simulink model "acc_num6"  (R2020a)
settings: Solver=ode4  StartTime=0.0  StopTime=endt  FixedStep=0.002  RelTol=1e-3  EnableMultiTasking=on
values from neighbouring files (symbols this model uses):
  Dy = 0.0085    [acc_parameter_num6.m]
  Jy = J_body + 2*J_prop + J_yoke    (= 0.0219920648283)    [acc_parameter_num6.m]
  K_A = 30    [acc_parameter_num6.m]
  K_B = 300    [acc_parameter_num6.m]
  Kd = 10    [acc_parameter_num6.m]
  lead_id = [1,2]    [acc_parameter_num6.m]
  pos_base = [x0;y0]    [acc_parameter_num6.m]
  psi_initial = [pi*3/4,pi/4,pi/4,pi/4,pi*5/6,pi*4/5]    [acc_parameter_num6.m]
  target = [10;33]    [acc_parameter_num6.m]
libraries: simulink_extras x6, aerolibanimutils x1, dspnetwork x1
settings Model: ExtModeTrigDuration=10000  Creator=Aline  LastModifiedBy=Aline
settings SolverCC: PositivePriorityOrder=on
settings DataIOCC: ReturnWorkspaceOutputs=off
settings OptimizationCC: LifeSpan=inf
settings DebuggingCC: ArithmeticOperatorsInVariantConditions=warning
settings SFSimCC: SimUseLocalCustomCode=off  CustomCodeUndefinedFunction=UseInterfaceOnly
settings RTWCC: Description=QUARC Win64 Target  SystemTargetFile=quarc_win64.tlc  TemplateMakefile=quarc_default_tmf  RTWUseLocalCustomCode=off
settings CodeAppCC: StateflowObjectComments=on
settings STFCustomTargetCC: TargetPreCompLibLocation=C:\PROGRA~3\QUARC\lib\2020a\win64\release  TargetLangStandard=C99 (ISO)  ConcurrentExecutionCompliant=on  GRTInterface=on  SystemTargetFile=quarc_win64.tlc
settings GRTTargetCC: TargetPreCompLibLocation=C:\PROGRA~3\QUARC\lib\2020a\win64\release  ParMdlRefBuildCompliant=off  CompOptLevelCompliant=off  CombineOutputUpdateFcns=off  MatFileLogging=off  CPPClassGenCompliant=off  GRTInterface=on  UseToolchainInfoCompliant=off  ExtMode=on  ExtModeMexFile=quarc_comm
settings ConfigComp: CovMetricSettings=dswe

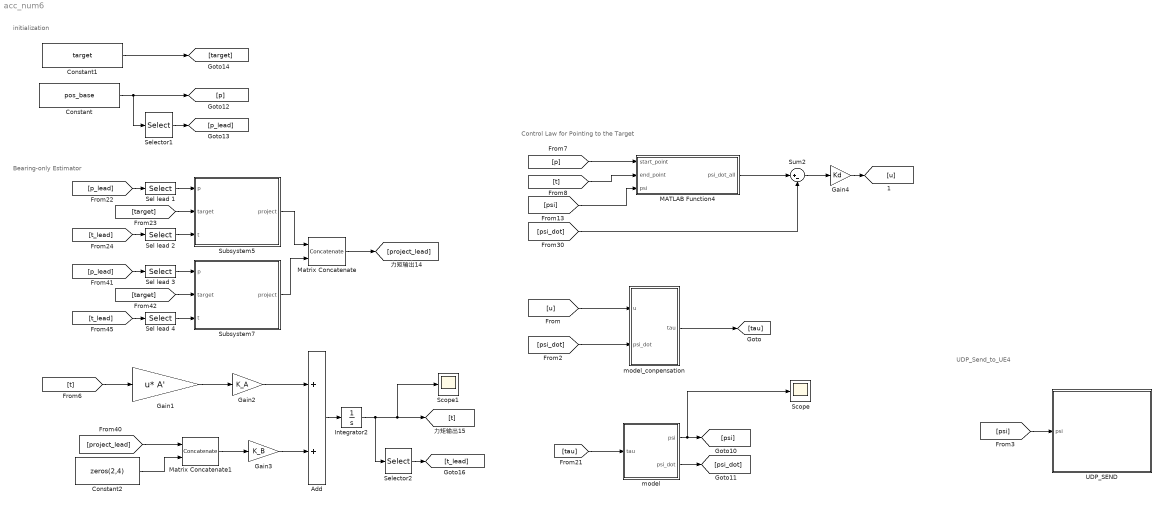
== system acc_num6 ==
  note: initialization
  note: Control Law for Pointing to the Target
  note: Bearing-only Estimator
  note: UDP_Send_to_UE4
  Add : Sum
  Constant : Constant  Value=pos_base
  Constant1 : Constant  Value=target  VectorParams1D=off
  Constant2 : Constant  Value=zeros(2,4)
  Gain1 : Gain  Gain=A'  Multiplication=Matrix(u*K)
  Gain2 : Gain  Gain=K_A
  Gain3 : Gain  Gain=K_B
  Gain4 : Gain  Gain=Kd
  Integrator2 : Integrator  InitialCondition=pos_base+ones(2,6)
  MATLAB Function4 : MATLAB Function  TreatAsAtomicUnit=on
  Matrix Concatenate : Concatenate  Mode=Multidimensional array  ConcatenateDimension=2
  Matrix Concatenate1 : Concatenate  Mode=Multidimensional array  ConcatenateDimension=2
  Scope : Scope
  Scope1 : Scope
  Sel lead 1 : Selector  NumberOfDimensions=2  InputPortWidth=3  IndexOptions=Index vector (dialog),Index vector (dialog)  Indices=[1 2],1  OutputSizes=1,1
  Sel lead 2 : Selector  NumberOfDimensions=2  InputPortWidth=3  IndexOptions=Index vector (dialog),Index vector (dialog)  Indices=[1 2],1  OutputSizes=1,1
  Sel lead 3 : Selector  NumberOfDimensions=2  InputPortWidth=3  IndexOptions=Index vector (dialog),Index vector (dialog)  Indices=[1 2],2  OutputSizes=1,1
  Sel lead 4 : Selector  NumberOfDimensions=2  InputPortWidth=3  IndexOptions=Index vector (dialog),Index vector (dialog)  Indices=[1 2],2  OutputSizes=1,1
  Selector1 : Selector  NumberOfDimensions=2  InputPortWidth=3  IndexOptions=Index vector (dialog),Index vector (dialog)  Indices=[1 2],lead_id  OutputSizes=1,1
  Selector2 : Selector  NumberOfDimensions=2  InputPortWidth=3  IndexOptions=Index vector (dialog),Index vector (dialog)  Indices=[1 2],lead_id  OutputSizes=1,1
  Subsystem5 : Subsystem
  Subsystem7 : Subsystem
  Sum2 : Sum  Inputs=|+-
  UDP_SEND : Subsystem
  model : Subsystem
  model_conpensation : Subsystem
  wires:
  [target] -> Subsystem5/2(target)
  Add/1 -> Integrator2/1
  Selector2/1 -> [t_lead]
  Gain1/1 -> Gain2/1
  Integrator2/1 -> Selector2/1, Scope1/1, [t]
  [t_lead] -> Sel lead 2/1
  [p_lead] -> Sel lead 1/1
  Sel lead 1/1 -> Subsystem5/1(p)
  Sel lead 2/1 -> Subsystem5/3(t)
  Sel lead 4/1 -> Subsystem7/3(t)
  [p_lead] -> Sel lead 3/1
  [t_lead] -> Sel lead 4/1
  [target] -> Subsystem7/2(target)
  Sel lead 3/1 -> Subsystem7/1(p)
  Constant/1 -> Selector1/1, [p]
  Gain3/1 -> Add/2
  Subsystem7/1(project) -> Matrix Concatenate/2
  Selector1/1 -> [p_lead]
  Subsystem5/1(project) -> Matrix Concatenate/1
  Matrix Concatenate/1 -> [project_lead]
  Constant1/1 -> [target]
  [project_lead] -> Matrix Concatenate1/1
  Constant2/1 -> Matrix Concatenate1/2
  Matrix Concatenate1/1 -> Gain3/1
  [u] -> model_conpensation/1(u)
  model/2(psi_dot) -> [psi_dot]
  model/1(psi) -> Scope/1, [psi]
  model_conpensation/1(tau) -> [tau]
  [psi] -> UDP_SEND/1(psi)
  [t] -> MATLAB Function4/2(end_point)
  [p] -> MATLAB Function4/1(start_point)
  Sum2/1 -> Gain4/1
  Gain4/1 -> [u]
  [tau] -> model/1(tau)
  [psi] -> MATLAB Function4/3(psi)
  [psi_dot] -> model_conpensation/2(psi_dot)
  [psi_dot] -> Sum2/2
  MATLAB Function4/1(psi_dot_all) -> Sum2/1
  [t] -> Gain1/1
  Gain2/1 -> Add/1

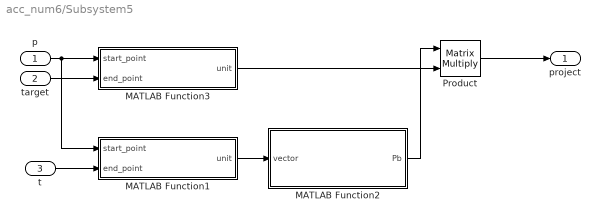
== system acc_num6/Subsystem5 ==
  p : Inport
  target : Inport  Port=2
  t : Inport  Port=3
  MATLAB Function1 : MATLAB Function  TreatAsAtomicUnit=on
  MATLAB Function2 : MATLAB Function  TreatAsAtomicUnit=on
  MATLAB Function3 : MATLAB Function  TreatAsAtomicUnit=on
  Product : Product  Multiplication=Matrix(*)
  project : Outport
  wires:
  MATLAB Function3/1(unit) -> Product/2
  target/1 -> MATLAB Function3/2(end_point)
  p/1 -> MATLAB Function1/1(start_point), MATLAB Function3/1(start_point)
  MATLAB Function1/1(unit) -> MATLAB Function2/1(vector)
  t/1 -> MATLAB Function1/2(end_point)
  MATLAB Function2/1(Pb) -> Product/1
  Product/1 -> project/1

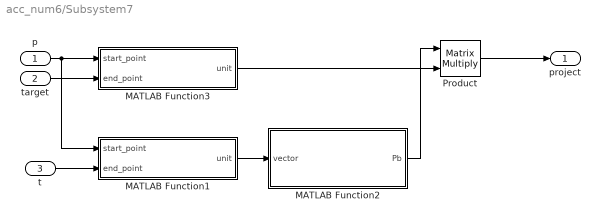
== system acc_num6/Subsystem7 ==
  p : Inport
  target : Inport  Port=2
  t : Inport  Port=3
  MATLAB Function1 : MATLAB Function  TreatAsAtomicUnit=on
  MATLAB Function2 : MATLAB Function  TreatAsAtomicUnit=on
  MATLAB Function3 : MATLAB Function  TreatAsAtomicUnit=on
  Product : Product  Multiplication=Matrix(*)
  project : Outport
  wires:
  Product/1 -> project/1
  MATLAB Function2/1(Pb) -> Product/1
  t/1 -> MATLAB Function1/2(end_point)
  MATLAB Function1/1(unit) -> MATLAB Function2/1(vector)
  p/1 -> MATLAB Function3/1(start_point), MATLAB Function1/1(start_point)
  target/1 -> MATLAB Function3/2(end_point)
  MATLAB Function3/1(unit) -> Product/2

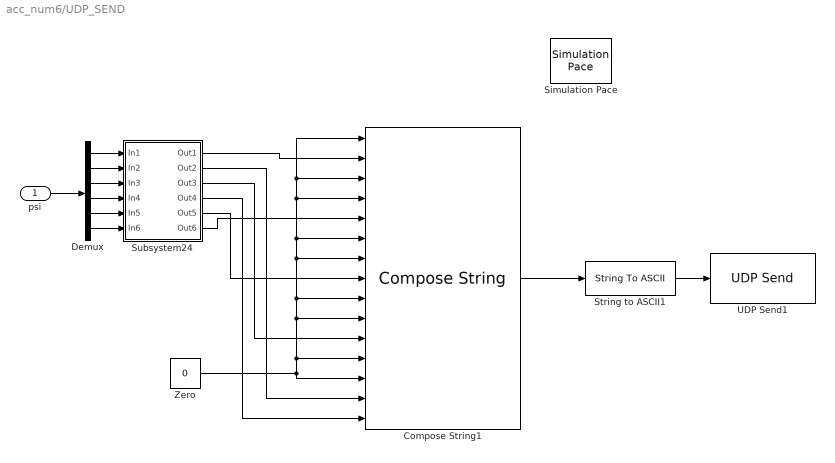
== system acc_num6/UDP_SEND ==
  psi : Inport
  Compose String1 : ComposeString  Format="\"pitch:%f;yaw:%f;roll:%f;pitch:%f;yaw:%f;roll:%f;pitch:%f;yaw:%f;roll:%f;pitch:%f;yaw:%f;roll:%f;pitch:%f;yaw:%f;roll:%f;\""
  Demux : Demux  Outputs=6
  Simulation Pace : aerolibanimutils/Simulation Pace  SimulationPace=1  SleepMode=Auto  OutputPaceError=off  SampleTime=0.1
  String to ASCII1 : StringToASCII  OutputVectorSize=225
  Subsystem24 : Subsystem
  UDP Send1 : dspnetwork/UDP Send  remoteURL='127.0.0.1'  remotePort=2333  localURL='0.0.0.0'  localPortSource=Automatically determine  localPort=-1  sendBufferSize=8192  sampletime=-1  blockPlatform=[]  separateLengthPort=0
  Zero : Constant  Value=0  OutDataTypeStr=Inherit: Inherit via back propagation
  wires:
  String to ASCII1/1 -> UDP Send1/1
  Subsystem24/6(Out6) -> Compose String1/5
  Demux/4 -> Subsystem24/4(In4)
  Compose String1/1 -> String to ASCII1/1
  Zero/1 -> Compose String1/13, Compose String1/1, Compose String1/3, Compose String1/4, Compose String1/6, Compose String1/7, Compose String1/9, Compose String1/10, Compose String1/12
  Demux/1 -> Subsystem24/1(In1)
  Subsystem24/3(Out3) -> Compose String1/11
  Subsystem24/4(Out4) -> Compose String1/15
  Subsystem24/1(Out1) -> Compose String1/2
  Subsystem24/5(Out5) -> Compose String1/8
  Demux/3 -> Subsystem24/3(In3)
  Subsystem24/2(Out2) -> Compose String1/14
  Demux/5 -> Subsystem24/5(In5)
  Demux/2 -> Subsystem24/2(In2)
  Demux/6 -> Subsystem24/6(In6)
  psi/1 -> Demux/1

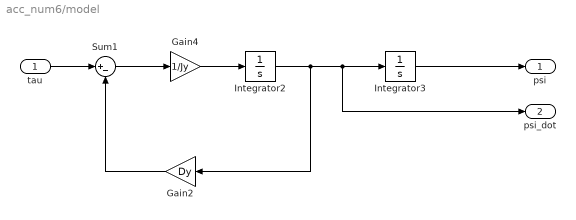
== system acc_num6/model ==
  tau : Inport
  Gain2 : Gain  Gain=Dy
  Gain4 : Gain  Gain=1/Jy
  Integrator2 : Integrator
  Integrator3 : Integrator  InitialCondition=psi_initial
  Sum1 : Sum  Inputs=|+-
  psi : Outport
  psi_dot : Outport  Port=2
  wires:
  Integrator2/1 -> Integrator3/1, psi_dot/1, Gain2/1
  Sum1/1 -> Gain4/1
  Gain4/1 -> Integrator2/1
  tau/1 -> Sum1/1
  Gain2/1 -> Sum1/2
  Integrator3/1 -> psi/1

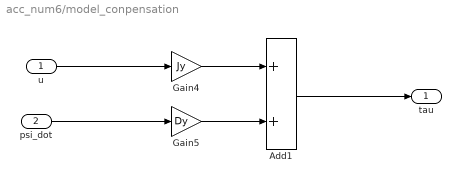
== system acc_num6/model_conpensation ==
  u : Inport
  psi_dot : Inport  Port=2
  Add1 : Sum
  Gain4 : Gain  Gain=Jy
  Gain5 : Gain  Gain=Dy
  tau : Outport
  wires:
  Gain4/1 -> Add1/1
  Gain5/1 -> Add1/2
  Add1/1 -> tau/1
  u/1 -> Gain4/1
  psi_dot/1 -> Gain5/1

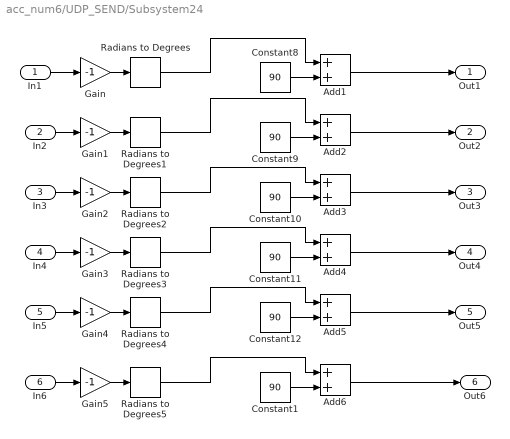
== system acc_num6/UDP_SEND/Subsystem24 ==
  In1 : Inport
  In2 : Inport  Port=2
  In3 : Inport  Port=3
  In4 : Inport  Port=4
  In5 : Inport  Port=5
  In6 : Inport  Port=6
  Add{1..6} (6 alike) : Sum
  Constant{1,8..12} (6 alike) : Constant  Value=90
  Gain{,1..5} (6 alike) : Gain  Gain=-1
  Radians to Degrees{,1..5} (6 alike) : simulink_extras/Transformations/Radians to Degrees
  Out1 : Outport
  Out2 : Outport  Port=2
  Out3 : Outport  Port=3
  Out4 : Outport  Port=4
  Out5 : Outport  Port=5
  Out6 : Outport  Port=6
  wires:
  Constant12/1 -> Add5/2
  In1/1 -> Gain/1
  Gain3/1 -> Radians to Degrees3/1
  Constant9/1 -> Add2/2
  Radians to Degrees2/1 -> Add3/1
  Add1/1 -> Out1/1
  In4/1 -> Gain3/1
  Constant8/1 -> Add1/2
  Constant10/1 -> Add3/2
  Radians to Degrees4/1 -> Add5/1
  Constant11/1 -> Add4/2
  Radians to Degrees3/1 -> Add4/1
  Gain1/1 -> Radians to Degrees1/1
  Add3/1 -> Out3/1
  Gain4/1 -> Radians to Degrees4/1
  Radians to Degrees/1 -> Add1/1
  Gain2/1 -> Radians to Degrees2/1
  Gain/1 -> Radians to Degrees/1
  Radians to Degrees1/1 -> Add2/1
  Add2/1 -> Out2/1
  In3/1 -> Gain2/1
  Add4/1 -> Out4/1
  In2/1 -> Gain1/1
  Add5/1 -> Out5/1
  In5/1 -> Gain4/1
  Gain5/1 -> Radians to Degrees5/1
  Radians to Degrees5/1 -> Add6/1
  Constant1/1 -> Add6/2
  In6/1 -> Gain5/1
  Add6/1 -> Out6/1

== matlab function acc_num6/Subsystem5/MATLAB Function1 ==
  data: start_point input; unit output; end_point input
function unit = unit_vector(start_point,end_point)
%给出向量的起点和终点 计算单位矢量
%start_point 向量起点       2*1
%end_point   向量终点       2*1
%unit        输出的单位向量 2*1
vector = end_point - start_point;
dist = sqrt(vector(1)^2+vector(2)^2);
if dist == 0
    unit = [0;0];
else
    unit = vector/dist;
end

== matlab function acc_num6/Subsystem5/MATLAB Function2 ==
  data: vector input; Pb output
function Pb = project_matrix(vector)
%正交投影矩阵
%vector 输入的单位向量 N*1
%Pb     输出的投影矩阵 N*N
%unit        输出的单位向量 2*1
size_v = size(vector,1);
Pb = eye(size_v) - vector*vector';
end

== matlab function acc_num6/Subsystem5/MATLAB Function3 ==
  data: start_point input; unit output; end_point input
function unit = unit_vector(start_point,end_point)
%给出向量的起点和终点 计算单位矢量
%start_point 向量起点       2*1
%end_point   向量终点       2*1
%unit        输出的单位向量 2*1
vector = end_point - start_point;
dist = sqrt(vector(1)^2+vector(2)^2);
if dist == 0
    unit = [0;0];
else
    unit = vector/dist;
end

== matlab function acc_num6/Subsystem7/MATLAB Function1 ==
  data: start_point input; unit output; end_point input
function unit = unit_vector(start_point,end_point)
%给出向量的起点和终点 计算单位矢量
%start_point 向量起点       2*1
%end_point   向量终点       2*1
%unit        输出的单位向量 2*1
vector = end_point - start_point;
dist = sqrt(vector(1)^2+vector(2)^2);
if dist == 0
    unit = [0;0];
else
    unit = vector/dist;
end

== matlab function acc_num6/Subsystem7/MATLAB Function2 ==
  data: vector input; Pb output
function Pb = project_matrix(vector)
%正交投影矩阵
%vector 输入的单位向量 N*1
%Pb     输出的投影矩阵 N*N
%unit        输出的单位向量 2*1
size_v = size(vector,1);
Pb = eye(size_v) - vector*vector';
end

== matlab function acc_num6/Subsystem7/MATLAB Function3 ==
  data: start_point input; unit output; end_point input
function unit = unit_vector(start_point,end_point)
%给出向量的起点和终点 计算单位矢量
%start_point 向量起点       2*1
%end_point   向量终点       2*1
%unit        输出的单位向量 2*1
vector = end_point - start_point;
dist = sqrt(vector(1)^2+vector(2)^2);
if dist == 0
    unit = [0;0];
else
    unit = vector/dist;
end

== matlab function acc_num6/MATLAB Function4 ==
  data: start_point input; psi_dot_all output; end_point input; psi input
function psi_dot_all = unit(start_point,end_point,psi)
%给出向量的起点和终点 计算单位矢量
%start_point 向量起点       2*n
%end_point   向量终点       2*n
%psi        输出的单位向量  1*n  

vector1 = end_point(:,1) - start_point(:,1);
dist1 = sqrt(vector1(1)^2+vector1(2)^2);
unit1 = vector1/dist1;
psi_dot_1=[-sin(psi(1)),cos(psi(1))] * unit1

vector2 = end_point(:,2) - start_point(:,2);
dist2 = sqrt(vector2(1)^2+vector2(2)^2);
unit2 = vector2/dist2;
psi_dot_2=[-sin(psi(2)),cos(psi(2))]*unit2

vector3 = end_point(:,3) - start_point(:,3);
dist3 = sqrt(vector3(1)^2+vector3(2)^2);
unit3 = vector3/dist3;
psi_dot_3=[-sin(psi(3)),cos(psi(3))]*unit3

vector4 = end_point(:,4) - start_point(:,4);
dist4 = sqrt(vector4(1)^2+vector4(2)^2);
unit4 = vector4/dist4;
psi_dot_4=[-sin(psi(4)),cos(psi(4))]*unit4

vector5 = end_point(:,5) - start_point(:,5);
dist5 = sqrt(vector5(1)^2+vector5(2)^2);
unit5 = vector5/dist5;
psi_dot_5=[-sin(psi(5)),cos(psi(5))]*unit5

vector6 = end_point(:,6) - start_point(:,6);
dist6 = sqrt(vector6(1)^2+vector6(2)^2);
unit6 = vector6/dist6;
psi_dot_6=[-sin(psi(6)),cos(psi(6))]*unit6

unit_all=[unit1,unit2,unit3,unit4,unit5,unit6];
psi_dot_all=[psi_dot_1,psi_dot_2,psi_dot_3,psi_dot_4,psi_dot_5,psi_dot_6]

% num=size(start_point,2);
% unit_all=[];
% for i = 1:num
% vector = end_point(:,i) - start_point(:,i);
% dist = sqrt(vector(1)^2+vector(2)^2);
% unit = vector/dist;
% unit_all=[unit_all,unit];
% end
% matrix_psi_dot=[-sin(psi);cos(psi)]'*unit_all
% psi_dot=diag(matrix_psi_dot)
